simulink model "Raspi"  (R2021b)
settings: Solver=FixedStepDiscrete  StartTime=0.0  StopTime=inf  FixedStep=1e-4  RelTol=1e-3  EnableMultiTasking=on
libraries: raspberrypiNetworklib x2
settings Model: SimulationMode=external  Creator=Blade  LastModifiedBy=Blade
settings SolverCC: PositivePriorityOrder=on
settings OptimizationCC: EnhancedBackFolding=on  PassReuseOutputArgsAs=Individual arguments  ZeroExternalMemoryAtStartup=off  ZeroInternalMemoryAtStartup=off  MaxStackSize=64  OptimizeBlockOrder=speed  DifferentSizesBufferReuse=on  OptimizationCustomize=off  EfficientTunableParamExpr=on
settings DebuggingCC: ParameterTunabilityLossMsg=error  UnderSpecifiedDimensionMsg=warning
settings HardwareCC: ProdBitPerPointer=32  ProdBitPerSizeT=32  ProdBitPerPtrDiffT=32  ProdLargestAtomicInteger=Long  ProdLargestAtomicFloat=Double  ProdWordSize=32  ProdLongLongMode=on  ProdHWDeviceType=ARM Compatible->ARM Cortex
settings RTWCC: Description=Embedded Coder  SystemTargetFile=ert.tlc  HardwareBoard=Raspberry Pi  TLCOptions="-aInlineSetEventsForThisBaseRateFcn=TLC_FALSE -aSuppressMultiTaskScheduler=TLC_FALSE  -aRateBasedStepFcn=0"  TemplateMakefile=ert_default_tmf  Toolchain=GNU GCC Embedded Linux  BuildConfiguration=Faster Runs
settings CodeAppCC: ForceParamTrailComments=on  IgnoreCustomStorageClasses=off  OperatorAnnotations=on  SimulinkDataObjDesc=on  SFDataObjDesc=on  InsertBlockDesc=on
settings ERTTargetCC: SupportContinuousTime=on  SupportVariableSizeSignals=on  ExtModeTransport=2  ExtModeStaticAlloc=on  ExtModeMexFile=ext_xcp  ExtModeIntrfLevel=Level2 - Open

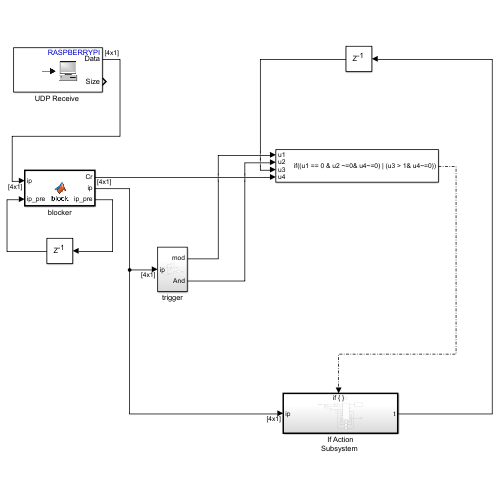
[thumbnail: Simulink's stored preview of the top-level diagram]
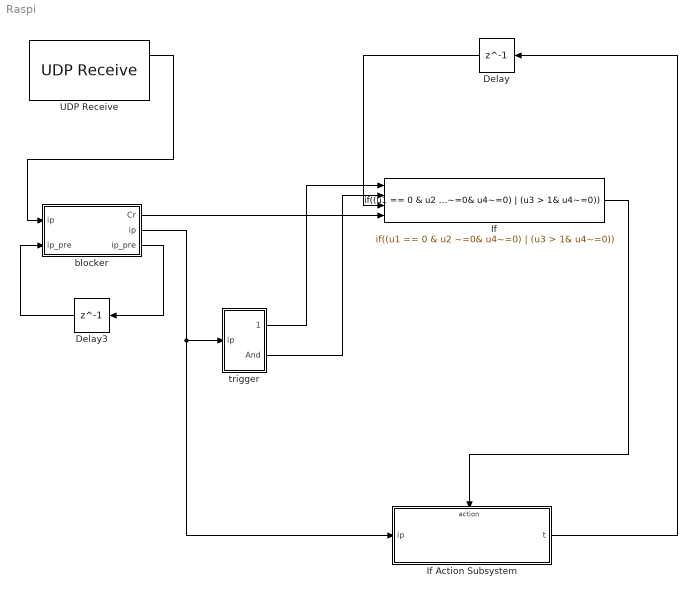
== system Raspi ==
  Delay : Delay  DelayLength=1  InitialCondition=0
  Delay3 : Delay  DelayLength=1  InitialCondition=0
  If : If  NumInputs=4  IfExpression=(u1 == 0 & u2 ~=0& u4~=0) | (u3 > 1& u4~=0)  ShowElse=off
  "If Action Subsystem " : Subsystem  TreatAsAtomicUnit=on
  "UDP Receive " : raspberrypiNetworklib/UDP Receive  localURL='0.0.0.0'  localPort=1000  remoteURL='0.0.0.0'  remotePort=-1  recvBufferSize=8192  signalDatatype=double  dims=4  isVarSize=off  showBlockingTime=off  blockingTime=0  sampletime=-1  blockPlatform=Raspberry Pi
      settings: SourceProductBaseCode=RASPPI
  blocker : MATLAB Function  TreatAsAtomicUnit=on
  trigger : Subsystem
  wires:
  blocker/2(ip) -> "If Action Subsystem "/1(ip), trigger/1(ip)
  trigger/2(And) -> If/2
  Delay/1 -> If/3
  trigger/1(mod) -> If/1
  "If Action Subsystem "/1(t) -> Delay/1
  Delay3/1 -> blocker/2("ip_pre ")
  "UDP Receive "/1 -> blocker/1("ip ")
  blocker/3(ip_pre) -> Delay3/1
  blocker/1(Cr) -> If/4
  If/1 -> "If Action Subsystem "/Action

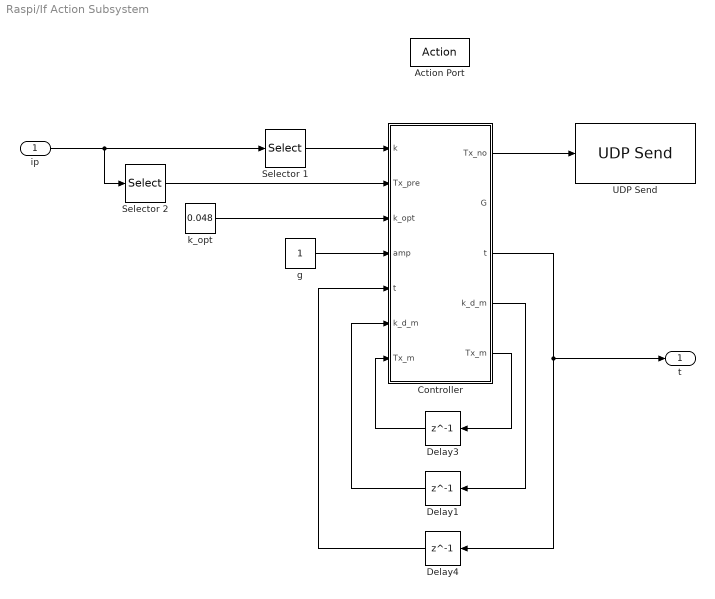
== system Raspi/If Action Subsystem  ==
  ip : Inport
  Action Port : ActionPort  ActionPortLabel=if((u1 == 0 & u2 ~=0& u4~=0) | (u3 > 1& u4~=0))
  Controller : MATLAB Function  TreatAsAtomicUnit=on
  Delay1 : Delay  DelayLength=1  InitialCondition=zeros(2,3)
  Delay3 : Delay  DelayLength=1  InitialCondition=zeros(8,2)
  Delay4 : Delay  DelayLength=1  InitialCondition=0
  Selector 1 : Selector  InputPortWidth=4  IndexOptions=Index vector (dialog)  Indices=1  OutputSizes=1
  Selector 2 : Selector  InputPortWidth=4  IndexOptions=Index vector (dialog)  Indices=[3;4]  OutputSizes=1
  "UDP Send " : raspberrypiNetworklib/UDP Send  remoteURL='172.20.10.2'  remotePort=2000  localURL='0.0.0.0'  localPortSource=Automatically determine  localPort=-1  sampletime=-1  blockPlatform=Raspberry Pi  separateLengthPort=0
      settings: SourceProductBaseCode=RASPPI
  g : Constant
  k_opt : Constant  Value=0.048
  t : Outport
  wires:
  Controller/5(Tx_m) -> Delay3/1
  Controller/4(k_d_m) -> Delay1/1
  Delay1/1 -> Controller/6("k_d_m ")
  Selector 1/1 -> Controller/1(k)
  Controller/3(t) -> Delay4/1, t/1
  Delay4/1 -> Controller/5("t ")
  Controller/1(Tx_no) -> "UDP Send "/1
  g/1 -> Controller/4(amp)
  Selector 2/1 -> Controller/2(Tx_pre)
  Delay3/1 -> Controller/7("Tx_m ")
  ip/1 -> Selector 2/1, Selector 1/1
  k_opt/1 -> Controller/3(k_opt)

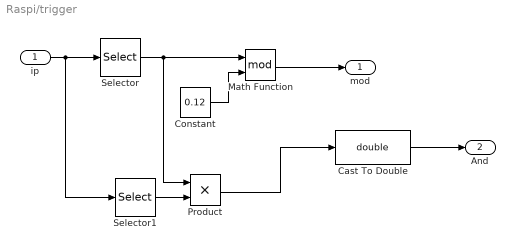
== system Raspi/trigger ==
  ip : Inport
  Cast To Double : DataTypeConversion  OutDataTypeStr=double
  Constant : Constant  Value=0.12
  Math Function : Math  Operator=mod  SaturateOnIntegerOverflow=on
  Product : Product
  Selector : Selector  InputPortWidth=4  IndexOptions=Index vector (dialog)  Indices=2  OutputSizes=1
  Selector1 : Selector  InputPortWidth=4  IndexOptions=Index vector (dialog)  Indices=1  OutputSizes=1
  mod : Outport
  And : Outport  Port=2
  wires:
  Constant/1 -> Math Function/2
  Selector/1 -> Product/1, Math Function/1
  ip/1 -> Selector1/1, Selector/1
  Math Function/1 -> mod/1
  Product/1 -> Cast To Double/1
  Selector1/1 -> Product/2
  Cast To Double/1 -> And/1

== matlab function Raspi/blocker ==
  data: Cr output; ip output; ip input; ip_pre input; ip_pre output
function [Cr,ip, ip_pre] = block(ip, ip_pre)

ip2 = ip(2);

if ip2 == ip_pre
    Cr = 0;
else
    ip_pre = ip2;
    Cr = 1;

end

== matlab function Raspi/If Action Subsystem /Controller ==
  data: k input; Tx_pre input; Tx_no output; G output; t output; k_opt input; amp input; t input; k_d_m output; k_d_m input; Tx_m input; Tx_m output
function [Tx_no,G,t,k_d_m,Tx_m] = Controller(k,Tx_pre,k_opt,amp,t,k_d_m,Tx_m)

k_diff = abs(k_opt-k)/k_opt;
Tx_pre = Tx_pre';

if t == 0
   

    t = t+1;
    k_d_m(1,:)  = [k_diff,Tx_pre];
    k_d_m(2,:)  = [k_diff,Tx_pre];

    
else

    if k_diff < k_d_m(2,1)

       k_d_m(2,:)  = [k_diff,Tx_pre];

    end

end

G = round(amp*k_d_m(1,1));  
Tx_fix = k_d_m(1,2:3)';

if t < 10
    if t < 9

        dir_att = [-1,-1; -1,0; 0,-1; 1,1; 1,0; 0,1; 1,-1; -1,1];
        
        
        Tx_no =G*dir_att(t,:)'+Tx_fix;
    
        Tx_m (t,:) = Tx_no;

    else

         Tx_no = k_d_m(2,2:3)'; % back to centre

    end

    t =t+1;

else
    
    
    Tx_no = k_d_m(2,2:3)';

    t =0;
   
 
end
